simulink model "gm_uz_pmsm_model_9ph_21b_all_double"  (R2021b)
settings: Solver=FixedStepDiscrete  StartTime=0.0  StopTime=0.8  RelTol=1e-3
PreLoadFcn:
  | uz_pmsm_model_9ph_init_parameter
undefined symbols (not defined in the file or in its folder): a, b, c, friction_coefficient, inertia, k_i_d, k_i_q, k_p_d, k_p_q, Kpd, L_d, L_o1, L_o2, L_q, L_x1, L_x2, L_y1, L_y2, L_zero, polepair, psi_pm, R_1, static_friction_torque, Tnd
libraries: hdlmdlgenlib x139, hdlsllib x90, dspsigops x21, simulink x3, slpidlib x2, spsAlphaBetaZerotodq0Lib x1, pid_lib x1, spsdq0toAlphaBetaZeroLib x1
(part 1 of 5)
settings Model: Creator=ts  LastModifiedBy=ts
settings SolverCC: AlgebraicLoopSolver=TrustRegion  AutoInsertRateTranBlk=on
settings DataIOCC: LimitDataPoints=on  SaveOutput=off  SaveTime=off
settings OptimizationCC: BlockReduction=off  ConditionallyExecuteInputs=off  DefaultParameterBehavior=Inlined  InheritOutputTypeSmallerThanSingle=on  LifeSpan=inf
settings DebuggingCC: AlgebraicLoopMsg=error  ArtificialAlgebraicLoopMsg=none  InheritedTsInSrcMsg=none  SingleTaskRateTransMsg=error  AllowSymbolicDim=off  StrictBusMsg=ErrorOnBusTreatedAsVector  SFUnexpectedBacktrackingDiag=warning  SFNoUnconditionalDefaultTransitionDiag=warning  SFExecutionAtInitializationDiag=none  SFMachineParentedDataDiag=warning  ArithmeticOperatorsInVariantConditions=warning
settings HardwareCC: ProdBitPerPointer=32  ProdBitPerSizeT=32  ProdBitPerPtrDiffT=32  ProdLargestAtomicFloat=None  ProdIntDivRoundTo=Undefined  ProdEndianess=Unspecified  ProdWordSize=32  ProdHWDeviceType=ASIC/FPGA->ASIC/FPGA  ProdEqTarget=off
settings SFSimCC: SimUseLocalCustomCode=off  CustomCodeUndefinedFunction=UseInterfaceOnly
settings RTWCC: RTWUseLocalCustomCode=off
settings CodeAppCC: StateflowObjectComments=on
settings GRTTargetCC: TargetLangStandard=C89/C90 (ANSI)
settings ConfigComp: CovScope=ReferencedModels  CovMetricSettings=dw  CovSaveCumulativeToWorkspaceVar=on  CovSaveSingleToWorkspaceVar=on  CovExternalEMLEnable=off  CovSFcnEnable=off

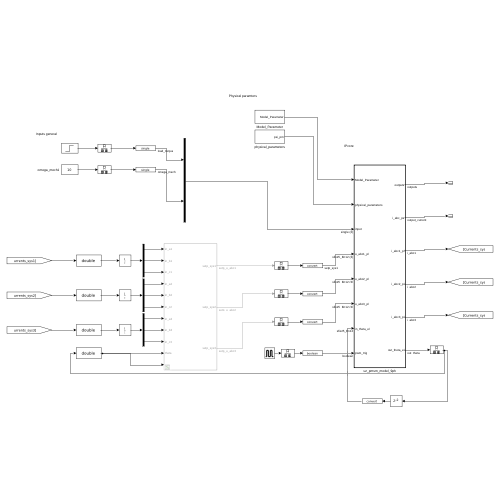
[thumbnail: Simulink's stored preview of the top-level diagram]
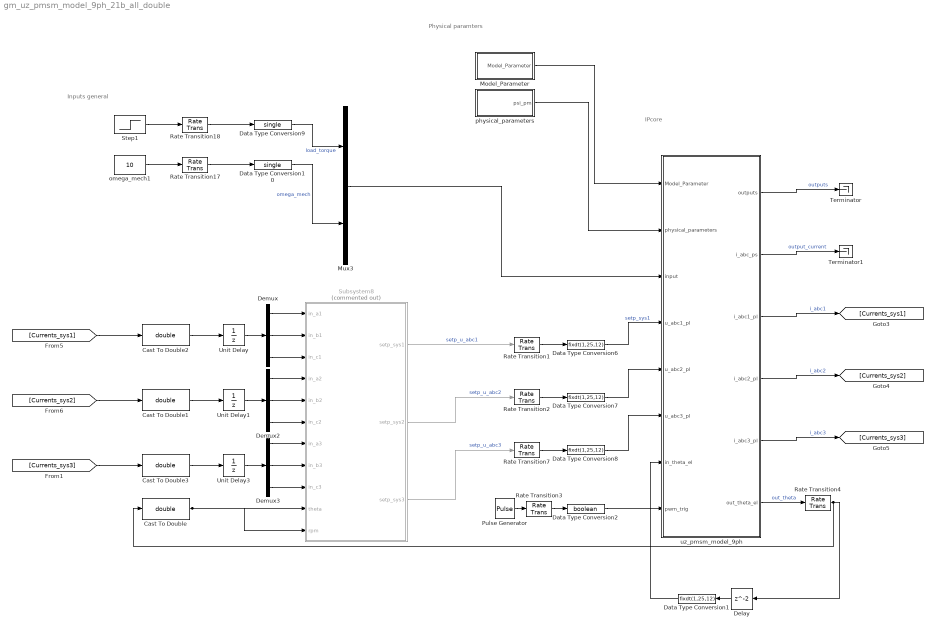
== system gm_uz_pmsm_model_9ph_21b_all_double ==
  note: Inputs general
  note: Physical paramters
  note: IPcore
  Cast To Double{,1..3} (4 alike) : DataTypeConversion  OutDataTypeStr=double
  Data Type Conversion{1,6..8} (4 alike) : DataTypeConversion  OutDataTypeStr=fixdt(1,25,12)  RndMeth=Nearest
  Data Type Conversion10 : DataTypeConversion  OutDataTypeStr=single  RndMeth=Nearest
  Data Type Conversion2 : DataTypeConversion  OutDataTypeStr=boolean  RndMeth=Nearest
  Data Type Conversion9 : DataTypeConversion  OutDataTypeStr=single  RndMeth=Nearest
  Delay : Delay
  Demux : Demux  Outputs=3
  Demux2 : Demux  Outputs=3
  Demux3 : Demux  Outputs=3
  Model_Parameter : Subsystem
  Mux3 : Mux  Inputs=2
  Pulse Generator : DiscretePulseGenerator  PulseType=Time based  Period=1e-9  PulseWidth=50
  Rate Transition{1..4,7,17..18} (7 alike) : RateTransition  OutPortSampleTime=ts
  Step1 : Step  Time=0.25  After=20  SampleTime=0
  Subsystem8 : Subsystem  Commented=on
  Terminator : Terminator
  Terminator1 : Terminator
  Unit Delay : UnitDelay  SampleTime=-1  HasFrameUpgradeWarning=on
  Unit Delay1 : UnitDelay  SampleTime=-1  HasFrameUpgradeWarning=on
  Unit Delay3 : UnitDelay  SampleTime=-1  HasFrameUpgradeWarning=on
  omega_mech1 : Constant  Value=10
  physical_parameters : Subsystem
  uz_pmsm_model_9ph : Subsystem  TreatAsAtomicUnit=on
  wires:
  Rate Transition4/1 -> Cast To Double/1, Delay/1
  Pulse Generator/1 -> Rate Transition3/1
  Rate Transition3/1 -> Data Type Conversion2/1
  Data Type Conversion2/1 -> uz_pmsm_model_9ph/8(pwm_trig)
  Rate Transition7/1 -> Data Type Conversion8/1
  Rate Transition2/1 -> Data Type Conversion7/1
  Rate Transition1/1 -> Data Type Conversion6/1
  Cast To Double3/1 -> Unit Delay3/1
  Cast To Double2/1 -> Unit Delay/1
  Cast To Double1/1 -> Unit Delay1/1
  Cast To Double/1 -> Subsystem8/10(theta), Subsystem8/11(rpm)
  Demux2/3 -> Subsystem8/6(in_c2)
  Demux2/2 -> Subsystem8/5(in_b2)
  Demux/1 -> Subsystem8/1(in_a1)
  Demux3/1 -> Subsystem8/7(in_a3)
  [Currents_sys3] -> Cast To Double3/1
  Unit Delay/1 -> Demux/1
  Demux3/3 -> Subsystem8/9(in_c3)
  [Currents_sys2] -> Cast To Double1/1
  [Currents_sys1] -> Cast To Double2/1
  Demux/3 -> Subsystem8/3(in_c1)
  Unit Delay1/1 -> Demux2/1
  Demux3/2 -> Subsystem8/8(in_b3)
  Demux2/1 -> Subsystem8/4(in_a2)
  Demux/2 -> Subsystem8/2(in_b1)
  Unit Delay3/1 -> Demux3/1
  Data Type Conversion7/1 -> uz_pmsm_model_9ph/5(u_abc2_pl)
  Data Type Conversion8/1 -> uz_pmsm_model_9ph/6(u_abc3_pl)
  Subsystem8/3(setp_sys3) -> Rate Transition7/1  "setp_u_abc3"
  Subsystem8/2(setp_sys2) -> Rate Transition2/1  "setp_u_abc2"
  Data Type Conversion6/1 -> uz_pmsm_model_9ph/4(u_abc1_pl)  "setp_sys1"
  Subsystem8/1(setp_sys1) -> Rate Transition1/1  "setp_u_abc1"
  Delay/1 -> Data Type Conversion1/1
  uz_pmsm_model_9ph/6(out_theta_el) -> Rate Transition4/1  "out_theta"
  uz_pmsm_model_9ph/4(i_abc2_pl) -> [Currents_sys2]  "i_abc2"
  uz_pmsm_model_9ph/5(i_abc3_pl) -> [Currents_sys3]  "i_abc3"
  uz_pmsm_model_9ph/3(i_abc1_pl) -> [Currents_sys1]  "i_abc1"
  uz_pmsm_model_9ph/2(i_abc_ps) -> Terminator1/1  "output_current"
  Data Type Conversion1/1 -> uz_pmsm_model_9ph/7(in_theta_el)
  Mux3/1 -> uz_pmsm_model_9ph/3(input)
  Data Type Conversion9/1 -> Mux3/1  "load_torque"
  Rate Transition17/1 -> Data Type Conversion10/1
  Data Type Conversion10/1 -> Mux3/2  "omega_mech"
  Step1/1 -> Rate Transition18/1
  Rate Transition18/1 -> Data Type Conversion9/1
  omega_mech1/1 -> Rate Transition17/1
  Model_Parameter/1(Model_Parameter) -> uz_pmsm_model_9ph/1(Model_Parameter)
  uz_pmsm_model_9ph/1(outputs) -> Terminator/1  "outputs"
  physical_parameters/1(psi_pm) -> uz_pmsm_model_9ph/2(physical_parameters)

== system gm_uz_pmsm_model_9ph_21b_all_double/Model_Parameter ==
  note: This flag determines if omega_mech is used as an input value or
      | if the mechanical system is simulated by the model
  Bus Creator : BusCreator  Inputs=4
  Constant3 : Constant  Value=0
  Data Type Conversion{3..4,9..10} (4 alike) : DataTypeConversion  OutDataTypeStr=boolean
  Rate Transition{6,8,17..18} (4 alike) : RateTransition  OutPortSampleTime=ts
  simulate_mechanical : Constant  Value=false
  simulate_mechanical1 : Constant  Value=false
  simulate_mechanical2 : Constant  Value=false
  Model_Parameter : Outport
  wires:
  Data Type Conversion3/1 -> Bus Creator/1  "reset_integrators"
  Bus Creator/1 -> Model_Parameter/1
  Data Type Conversion4/1 -> Bus Creator/2  "simulate_mechanical"
  Data Type Conversion9/1 -> Bus Creator/3  "switch_pspl"
  Data Type Conversion10/1 -> Bus Creator/4  "control_dq_abc"
  Rate Transition18/1 -> Data Type Conversion10/1
  Rate Transition17/1 -> Data Type Conversion9/1
  simulate_mechanical1/1 -> Rate Transition17/1
  Constant3/1 -> Rate Transition6/1
  Rate Transition6/1 -> Data Type Conversion3/1
  Rate Transition8/1 -> Data Type Conversion4/1
  simulate_mechanical/1 -> Rate Transition8/1
  simulate_mechanical2/1 -> Rate Transition18/1

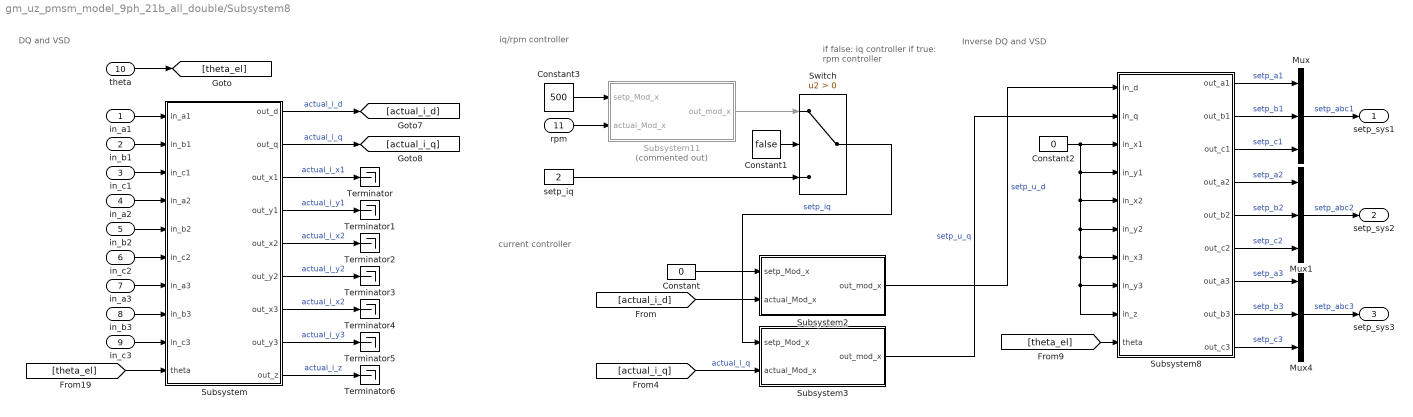
== system gm_uz_pmsm_model_9ph_21b_all_double/Subsystem8 ==
  note: Inverse DQ and VSD
  note: if false: iq controller
      | if true: rpm controller
  note: iq/rpm controller
  note: current controller
  note: DQ and VSD
  in_a1 : Inport
  in_b1 : Inport  Port=2
  in_c1 : Inport  Port=3
  in_a2 : Inport  Port=4
  in_b2 : Inport  Port=5
  in_c2 : Inport  Port=6
  in_a3 : Inport  Port=7
  in_b3 : Inport  Port=8
  in_c3 : Inport  Port=9
  theta : Inport  Port=10
  rpm : Inport  Port=11
  Constant : Constant  Value=0
  Constant1 : Constant  Value=false
  Constant2 : Constant  Value=0
  Constant3 : Constant  Value=500
  Mux : Mux  Inputs=3
  Mux1 : Mux  Inputs=3
  Mux4 : Mux  Inputs=3
  Subsystem : Subsystem
  Subsystem11 : Subsystem  Commented=on
  Subsystem2 : Subsystem
  Subsystem3 : Subsystem
  Subsystem8 : Subsystem
  Switch : Switch  Criteria=u2 > Threshold
  Terminator{,1..6} (7 alike) : Terminator
  setp_iq : Constant  Value=2
  setp_sys1 : Outport
  setp_sys2 : Outport  Port=2
  setp_sys3 : Outport  Port=3
  wires:
  Subsystem2/1(out_mod_x) -> Subsystem8/1(in_d)  "setp_u_d"
  Subsystem3/1(out_mod_x) -> Subsystem8/2(in_q)  "setp_u_q"
  Constant3/1 -> Subsystem11/1(setp_Mod_x)
  setp_iq/1 -> Switch/3
  Constant1/1 -> Switch/2
  Switch/1 -> Subsystem3/1(setp_Mod_x)  "setp_iq"
  Subsystem11/1(out_mod_x) -> Switch/1
  Constant2/1 -> Subsystem8/4(in_y1), Subsystem8/5(in_x2), Subsystem8/6(in_y2), Subsystem8/7(in_x3), Subsystem8/9(in_z), Subsystem8/8(in_y3), Subsystem8/3(in_x1)
  [theta_el] -> Subsystem/10(theta)
  Subsystem/2(out_q) -> [actual_i_q]  "actual_i_q"
  Subsystem/1(out_d) -> [actual_i_d]  "actual_i_d"
  rpm/1 -> Subsystem11/2(actual_Mod_x)
  Subsystem8/9(out_c3) -> Mux4/3  "setp_c3"
  Subsystem8/8(out_b3) -> Mux4/2  "setp_b3"
  Subsystem8/7(out_a3) -> Mux4/1  "setp_a3"
  Mux4/1 -> setp_sys3/1  "setp_abc3"
  Subsystem8/4(out_a2) -> Mux1/1  "setp_a2"
  Subsystem8/5(out_b2) -> Mux1/2  "setp_b2"
  Subsystem8/6(out_c2) -> Mux1/3  "setp_c2"
  Mux1/1 -> setp_sys2/1  "setp_abc2"
  in_a3/1 -> Subsystem/7(in_a3)
  in_b3/1 -> Subsystem/8(in_b3)
  in_c3/1 -> Subsystem/9(in_c3)
  Subsystem/9(out_z) -> Terminator6/1  "actual_i_z"
  Subsystem/7(out_x3) -> Terminator4/1  "actual_i_x2"
  Subsystem/8(out_y3) -> Terminator5/1  "actual_i_y3"
  Mux/1 -> setp_sys1/1  "setp_abc1"
  theta/1 -> [theta_el]
  in_c2/1 -> Subsystem/6(in_c2)
  in_a2/1 -> Subsystem/4(in_a2)
  in_b2/1 -> Subsystem/5(in_b2)
  [actual_i_q] -> Subsystem3/2(actual_Mod_x)  "actual_i_q"
  in_a1/1 -> Subsystem/1(in_a1)
  Subsystem/5(out_x2) -> Terminator2/1  "actual_i_x2"
  Subsystem/6(out_y2) -> Terminator3/1  "actual_i_y2"
  Constant/1 -> Subsystem2/1(setp_Mod_x)
  [actual_i_d] -> Subsystem2/2(actual_Mod_x)
  in_c1/1 -> Subsystem/3(in_c1)
  Subsystem/3(out_x1) -> Terminator/1  "actual_i_x1"
  Subsystem8/3(out_c1) -> Mux/3  "setp_c1"
  Subsystem8/2(out_b1) -> Mux/2  "setp_b1"
  [theta_el] -> Subsystem8/10(theta)
  in_b1/1 -> Subsystem/2(in_b1)
  Subsystem8/1(out_a1) -> Mux/1  "setp_a1"
  Subsystem/4(out_y1) -> Terminator1/1  "actual_i_y1"

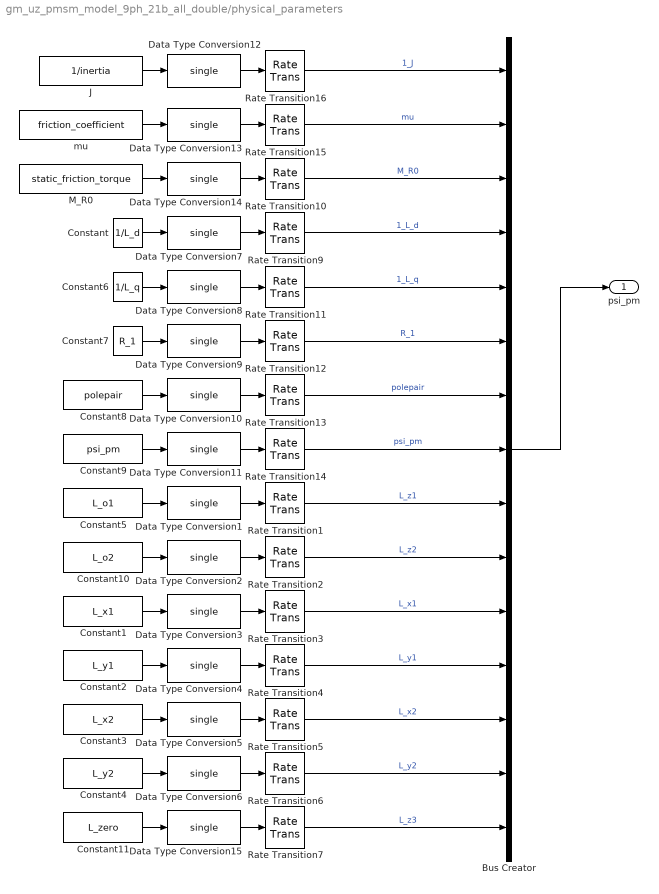
== system gm_uz_pmsm_model_9ph_21b_all_double/physical_parameters ==
  Bus Creator : BusCreator  Inputs=15
  Constant : Constant  Value=1/L_d
  Constant1 : Constant  Value=L_x1
  Constant10 : Constant  Value=L_o2
  Constant11 : Constant  Value=L_zero
  Constant2 : Constant  Value=L_y1
  Constant3 : Constant  Value=L_x2
  Constant4 : Constant  Value=L_y2
  Constant5 : Constant  Value=L_o1
  Constant6 : Constant  Value=1/L_q
  Constant7 : Constant  Value=R_1
  Constant8 : Constant  Value=polepair
  Constant9 : Constant  Value=psi_pm
  Data Type Conversion{1..15} (15 alike) : DataTypeConversion  OutDataTypeStr=single
  J : Constant  Value=1/inertia
  M_R0 : Constant  Value=static_friction_torque
  Rate Transition{1..7,9..16} (15 alike) : RateTransition  OutPortSampleTime=ts
  mu : Constant  Value=friction_coefficient
  psi_pm : Outport
  wires:
  Constant10/1 -> Data Type Conversion2/1
  Constant5/1 -> Data Type Conversion1/1
  Constant1/1 -> Data Type Conversion3/1
  Constant2/1 -> Data Type Conversion4/1
  Constant3/1 -> Data Type Conversion5/1
  Constant4/1 -> Data Type Conversion6/1
  Rate Transition2/1 -> Bus Creator/10  "L_z2"
  Rate Transition3/1 -> Bus Creator/11  "L_x1"
  Rate Transition4/1 -> Bus Creator/12  "L_y1"
  Rate Transition5/1 -> Bus Creator/13  "L_x2"
  Rate Transition6/1 -> Bus Creator/14  "L_y2"
  Rate Transition7/1 -> Bus Creator/15  "L_z3"
  Rate Transition1/1 -> Bus Creator/9  "L_z1"
  Data Type Conversion15/1 -> Rate Transition7/1
  Constant11/1 -> Data Type Conversion15/1
  Data Type Conversion6/1 -> Rate Transition6/1
  Data Type Conversion5/1 -> Rate Transition5/1
  Data Type Conversion4/1 -> Rate Transition4/1
  Data Type Conversion3/1 -> Rate Transition3/1
  Data Type Conversion2/1 -> Rate Transition2/1
  Data Type Conversion1/1 -> Rate Transition1/1
  Constant/1 -> Data Type Conversion7/1
  Constant9/1 -> Data Type Conversion11/1
  Constant7/1 -> Data Type Conversion9/1
  Data Type Conversion13/1 -> Rate Transition15/1
  Rate Transition11/1 -> Bus Creator/5  "1_L_q"
  M_R0/1 -> Data Type Conversion14/1
  mu/1 -> Data Type Conversion13/1
  Data Type Conversion10/1 -> Rate Transition13/1
  Data Type Conversion8/1 -> Rate Transition11/1
  J/1 -> Data Type Conversion12/1
  Rate Transition9/1 -> Bus Creator/4  "1_L_d"
  Constant6/1 -> Data Type Conversion8/1
  Rate Transition15/1 -> Bus Creator/2  "mu"
  Data Type Conversion9/1 -> Rate Transition12/1
  Constant8/1 -> Data Type Conversion10/1
  Data Type Conversion11/1 -> Rate Transition14/1
  Bus Creator/1 -> psi_pm/1
  Rate Transition13/1 -> Bus Creator/7  "polepair"
  Rate Transition16/1 -> Bus Creator/1  "1_J"
  Rate Transition12/1 -> Bus Creator/6  "R_1"
  Data Type Conversion14/1 -> Rate Transition10/1
  Rate Transition14/1 -> Bus Creator/8  "psi_pm"
  Rate Transition10/1 -> Bus Creator/3  "M_R0"
  Data Type Conversion7/1 -> Rate Transition9/1
  Data Type Conversion12/1 -> Rate Transition16/1

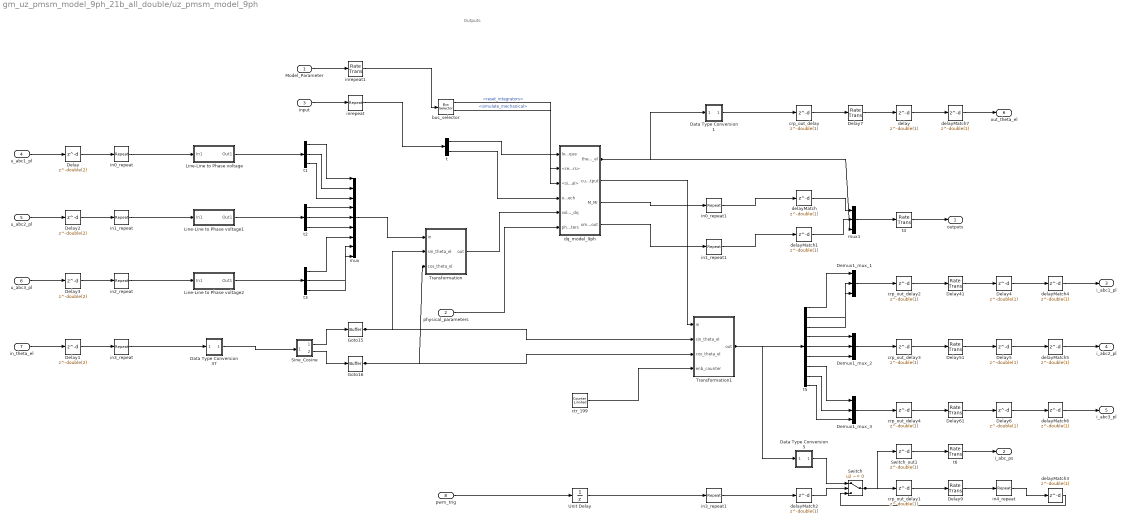
== system gm_uz_pmsm_model_9ph_21b_all_double/uz_pmsm_model_9ph ==
  note: Outputs
  Model_Parameter : Inport  SampleTime=2e-06
  physical_parameters : Inport  Port=2  SampleTime=2e-06
  input : Inport  Port=3  OutDataTypeStr=single  PortDimensions=[2]  SampleTime=2e-06
  u_abc1_pl : Inport  Port=4  OutDataTypeStr=fixdt(1, 25, 12)  PortDimensions=[3]  SampleTime=2e-06
  u_abc2_pl : Inport  Port=5  OutDataTypeStr=fixdt(1, 25, 12)  PortDimensions=[3]  SampleTime=2e-06
  u_abc3_pl : Inport  Port=6  OutDataTypeStr=fixdt(1, 25, 12)  PortDimensions=[3]  SampleTime=2e-06
  in_theta_el : Inport  Port=7  OutDataTypeStr=fixdt(1, 25, 12)  PortDimensions=1  SampleTime=2e-06
  pwm_trig : Inport  Port=8  OutDataTypeStr=boolean  PortDimensions=1  SampleTime=2e-06
  Data Type Conversion1 : Subsystem
      mask Display: disp('NFP\nconv');
  Data Type Conversion37 : Subsystem
      mask Display: disp('NFP\nconv');
  Data Type Conversion5 : Subsystem
      mask Display: disp('NFP\nconv');
  Delay{,1..3} (4 alike) : Delay  DelayLength=double(2)  InitialCondition=0  SampleTime=2e-06
  Delay4 : Delay  DelayLength=double(1)  InitialCondition=0  SampleTime=2e-06
  Delay{7,9,41,51,61} (5 alike) : RateTransition  OutPortSampleTimeOpt=Multiple of input port sample time  OutPortSampleTimeMultiple=200
  Delay5 : Delay  DelayLength=double(1)  InitialCondition=0  SampleTime=2e-06
  Delay6 : Delay  DelayLength=double(1)  InitialCondition=0  SampleTime=2e-06
  Demux1_mux_1 : Mux  Inputs=3
  Demux1_mux_2 : Mux  Inputs=3
  Demux1_mux_3 : Mux  Inputs=3
  Goto15 : hdlmdlgenlib/Buffer
      settings: SourceProductBaseCode=SL
  Goto16 : hdlmdlgenlib/Buffer
      settings: SourceProductBaseCode=SL
  Line-Line to Phase voltage : Subsystem
  Line-Line to Phase voltage1 : Subsystem
  Line-Line to Phase voltage2 : Subsystem
  Sine_Cosine : Subsystem
      mask Display: disp('NFP\ntrig2');
  Switch : Switch  Criteria=u2 ~= 0  Threshold=double(0)  OutDataTypeStr=single  SampleTime=1e-08
  Switch_out1 : Delay  DelayLength=double(1)  InitialCondition=0  SampleTime=1e-08
  Transformation : Subsystem
  Transformation1 : Subsystem
  Unit Delay : UnitDelay  SampleTime=2e-06
  bus_selector : BusSelector  OutputSignals=reset_integrators,simulate_mechanical
  crp_out_delay{,1..4} (5 alike) : Delay  DelayLength=double(1)  InitialCondition=0  SampleTime=1e-08
  ctr_199 : simulink/Sources/Counter Limited  uplimit=double(199)  tsamp=1e-08
  delay : Delay  DelayLength=double(1)  InitialCondition=0  SampleTime=2e-06
  delayMatch{,1..3} (4 alike) : Delay  DelayLength=double(1)  InitialCondition=0  SampleTime=1e-08
  delayMatch{4..7} (4 alike) : Delay  DelayLength=double(1)  InitialCondition=0  SampleTime=2e-06
  dq_model_9ph : Subsystem
  in0_repeat : dspsigops/Repeat  N=double(200)  RateOptions=Allow multirate processing  ic=0  mode=Unused parameter value
  in0_repeat1 : dspsigops/Repeat  N=double(200)  RateOptions=Allow multirate processing  ic=0  mode=Unused parameter value
  in1_repeat : dspsigops/Repeat  N=double(200)  RateOptions=Allow multirate processing  ic=0  mode=Unused parameter value
  in1_repeat1 : dspsigops/Repeat  N=double(200)  RateOptions=Allow multirate processing  ic=0  mode=Unused parameter value
  in2_repeat : dspsigops/Repeat  N=double(200)  RateOptions=Allow multirate processing  ic=0  mode=Unused parameter value
  in3_repeat : dspsigops/Repeat  N=double(200)  RateOptions=Allow multirate processing  ic=0  mode=Unused parameter value
  in3_repeat1 : dspsigops/Repeat  N=double(200)  RateOptions=Allow multirate processing  ic=0  mode=Unused parameter value
  in4_repeat : dspsigops/Repeat  N=double(200)  RateOptions=Allow multirate processing  ic=0  mode=Unused parameter value
  inrepeat : dspsigops/Repeat  N=double(200)  RateOptions=Allow multirate processing  ic=0  mode=Unused parameter value
  inrepeat1 : RateTransition  Integrity=off  Deterministic=off  OutPortSampleTimeOpt=Multiple of input port sample time  OutPortSampleTimeMultiple=1/200
  mux : Mux  Inputs=9
  mux1 : Mux  Inputs=3
  t : Demux  Outputs=2
  t1 : Demux  Outputs=3
  t2 : Demux  Outputs=3
  t3 : Demux  Outputs=3
  t4 : RateTransition  OutPortSampleTimeOpt=Multiple of input port sample time  OutPortSampleTimeMultiple=200
  t5 : Demux  Outputs=9
  t6 : RateTransition  OutPortSampleTimeOpt=Multiple of input port sample time  OutPortSampleTimeMultiple=200
  outputs : Outport  SampleTime=2e-06
  i_abc_ps : Outport  Port=2  SampleTime=2e-06
  i_abc1_pl : Outport  Port=3  SampleTime=2e-06
  i_abc2_pl : Outport  Port=4  SampleTime=2e-06
  i_abc3_pl : Outport  Port=5  SampleTime=2e-06
  out_theta_el : Outport  Port=6  SampleTime=2e-06
  wires:
  Model_Parameter/1 -> inrepeat1/1
  physical_parameters/1 -> dq_model_9ph/6(physical_parameters)
  input/1 -> inrepeat/1
  u_abc1_pl/1 -> Delay/1
  u_abc2_pl/1 -> Delay2/1
  u_abc3_pl/1 -> Delay3/1
  in_theta_el/1 -> Delay1/1
  pwm_trig/1 -> Unit Delay/1
  delayMatch7/1 -> out_theta_el/1
  Delay/1 -> in0_repeat/1
  Delay1/1 -> in3_repeat/1
  Delay2/1 -> in1_repeat/1
  Delay3/1 -> in2_repeat/1
  delayMatch4/1 -> i_abc1_pl/1
  delayMatch5/1 -> i_abc2_pl/1
  delayMatch6/1 -> i_abc3_pl/1
  Delay41/1 -> Delay4/1
  Delay51/1 -> Delay5/1
  Delay61/1 -> Delay6/1
  Unit Delay/1 -> in3_repeat1/1
  dq_model_9ph/3(M_Mi) -> in0_repeat1/1
  dq_model_9ph/4(omega_out) -> in1_repeat1/1
  Delay7/1 -> delay/1
  t/1 -> dq_model_9ph/1(load_torque)
  t/2 -> dq_model_9ph/4(omega_mech)
  bus_selector/1 -> dq_model_9ph/2(<reset_integrators>)  "<reset_integrators>"
  bus_selector/2 -> dq_model_9ph/3(<simulate_mechanical>)  "<simulate_mechanical>"
  Goto15/1 -> Transformation/2(sin_theta_el), Transformation1/2(sin_theta_el)
  Goto16/1 -> Transformation/3(cos_theta_el), Transformation1/3(cos_theta_el)
  Transformation/1(out) -> dq_model_9ph/5(voltage_input_dq)
  dq_model_9ph/1(theta_el) -> mux1/3, Data Type Conversion1/1(In1)
  dq_model_9ph/2(currents_dq_output) -> Transformation1/1(in)
  t4/1 -> outputs/1
  t6/1 -> i_abc_ps/1
  Delay4/1 -> delayMatch4/1
  Delay5/1 -> delayMatch5/1
  Delay6/1 -> delayMatch6/1
  delay/1 -> delayMatch7/1
  Delay9/1 -> in4_repeat/1
  inrepeat/1 -> t/1
  inrepeat1/1 -> bus_selector/1
  in0_repeat/1 -> Line-Line to Phase voltage/1(In1)
  in1_repeat/1 -> Line-Line to Phase voltage1/1(In1)
  in2_repeat/1 -> Line-Line to Phase voltage2/1(In1)
  in3_repeat/1 -> Data Type Conversion37/1(In1)
  Line-Line to Phase voltage/1(Out1) -> t1/1
  Line-Line to Phase voltage1/1(Out1) -> t2/1
  Line-Line to Phase voltage2/1(Out1) -> t3/1
  t1/1 -> mux/1
  t1/2 -> mux/2
  t1/3 -> mux/3
  t2/1 -> mux/4
  t2/2 -> mux/5
  t2/3 -> mux/6
  t3/1 -> mux/7
  t3/2 -> mux/8
  t3/3 -> mux/9
  Data Type Conversion37/1(Out1) -> Sine_Cosine/1(In1)
  Sine_Cosine/1(Out1) -> Goto15/1
  Sine_Cosine/2(Out2) -> Goto16/1
  mux/1 -> Transformation/1(in)
  mux1/1 -> t4/1
  in0_repeat1/1 -> delayMatch/1
  in1_repeat1/1 -> delayMatch1/1
  delayMatch/1 -> mux1/1
  delayMatch1/1 -> mux1/2
  crp_out_delay/1 -> Delay7/1
  Data Type Conversion1/1(Out1) -> crp_out_delay/1
  Switch_out1/1 -> t6/1
  crp_out_delay1/1 -> Delay9/1
  crp_out_delay2/1 -> Delay41/1
  crp_out_delay3/1 -> Delay51/1
  crp_out_delay4/1 -> Delay61/1
  in3_repeat1/1 -> delayMatch2/1
  in4_repeat/1 -> delayMatch3/1
  Transformation1/1(out) -> Data Type Conversion5/1(In1), t5/1
  t5/1 -> Demux1_mux_1/1
  t5/2 -> Demux1_mux_1/2
  t5/3 -> Demux1_mux_1/3
  t5/4 -> Demux1_mux_2/1
  t5/5 -> Demux1_mux_2/2
  t5/6 -> Demux1_mux_2/3
  t5/7 -> Demux1_mux_3/1
  t5/8 -> Demux1_mux_3/2
  t5/9 -> Demux1_mux_3/3
  delayMatch2/1 -> Switch/2
  delayMatch3/1 -> Switch/3
  Data Type Conversion5/1(Out1) -> Switch/1
  Demux1_mux_1/1 -> crp_out_delay2/1
  Demux1_mux_2/1 -> crp_out_delay3/1
  Demux1_mux_3/1 -> crp_out_delay4/1
  Switch/1 -> crp_out_delay1/1, Switch_out1/1
  ctr_199/1 -> Transformation1/4(enb_counter)

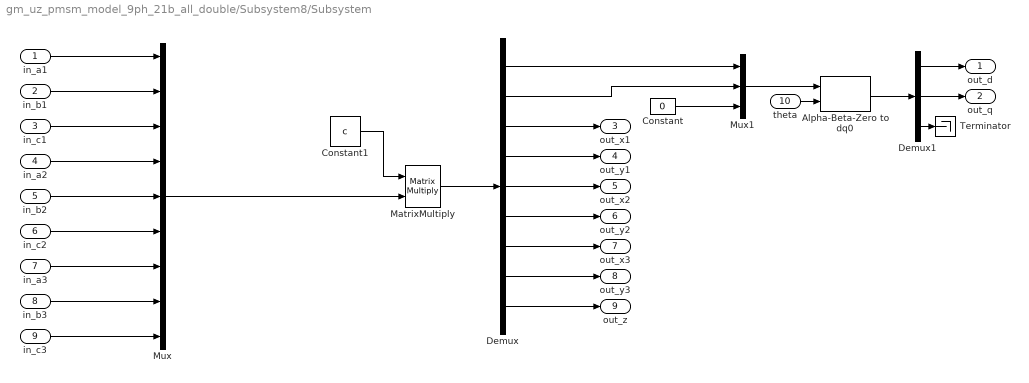
== system gm_uz_pmsm_model_9ph_21b_all_double/Subsystem8/Subsystem ==
  in_a1 : Inport
  in_b1 : Inport  Port=2
  in_c1 : Inport  Port=3
  in_a2 : Inport  Port=4
  in_b2 : Inport  Port=5
  in_c2 : Inport  Port=6
  in_a3 : Inport  Port=7
  in_b3 : Inport  Port=8
  in_c3 : Inport  Port=9
  theta : Inport  Port=10
  Alpha-Beta-Zero to dq0 : spsAlphaBetaZerotodq0Lib/Alpha-Beta-Zero to dq0  Alignment=90 degrees behind phase A axis
      settings: SourceProductBaseCode=PS
  Constant : Constant  Value=0
  Constant1 : Constant  Value=c
  Demux : Demux  Outputs=9
  Demux1 : Demux  Outputs=3
  MatrixMultiply : Product  Multiplication=Matrix(*)
  Mux : Mux  Inputs=9
  Mux1 : Mux  Inputs=3
  Terminator : Terminator
  out_d : Outport
  out_q : Outport  Port=2
  out_x1 : Outport  Port=3
  out_y1 : Outport  Port=4
  out_x2 : Outport  Port=5
  out_y2 : Outport  Port=6
  out_x3 : Outport  Port=7
  out_y3 : Outport  Port=8
  out_z : Outport  Port=9
  wires:
  in_b3/1 -> Mux/8
  in_a3/1 -> Mux/7
  in_c2/1 -> Mux/6
  in_b2/1 -> Mux/5
  in_a2/1 -> Mux/4
  in_c1/1 -> Mux/3
  in_b1/1 -> Mux/2
  Mux/1 -> MatrixMultiply/2
  Constant1/1 -> MatrixMultiply/1
  Alpha-Beta-Zero to dq0/1 -> Demux1/1
  Constant/1 -> Mux1/3
  Demux1/2 -> out_q/1
  Demux1/1 -> out_d/1
  Demux/2 -> Mux1/2
  Mux1/1 -> Alpha-Beta-Zero to dq0/1
  Demux/1 -> Mux1/1
  Demux1/3 -> Terminator/1
  theta/1 -> Alpha-Beta-Zero to dq0/2
  Demux/9 -> out_z/1
  Demux/8 -> out_y3/1
  Demux/7 -> out_x3/1
  in_c3/1 -> Mux/9
  Demux/3 -> out_x1/1
  MatrixMultiply/1 -> Demux/1
  Demux/5 -> out_x2/1
  in_a1/1 -> Mux/1
  Demux/4 -> out_y1/1
  Demux/6 -> out_y2/1

== system gm_uz_pmsm_model_9ph_21b_all_double/Subsystem8/Subsystem11 ==
  setp_Mod_x : Inport
  actual_Mod_x : Inport  Port=2
  Add : Sum  Inputs=+-
  Data Type Conversion8 : DataTypeConversion  OutDataTypeStr=double
  PID Controller2 : pid_lib/PID Controller  Controller=PI  Form=Ideal  TimeDomain=Continuous-time  UseExternalTs=off  SampleTime=-1  IntegratorMethod=Forward Euler  FilterMethod=Forward Euler  ControllerParametersSource=internal  P=Kpd  I=1/Tnd  D=0  N=100  UseFilter=on  TunerSelectOption=Transfer Function Based (PID Tuner App)  InitialConditionSource=internal  InitialConditionForIntegrator=0  InitialConditionForFilter=0  DifferentiatorICPrevScaledInput=0  ExternalReset=none  TrackingMode=off  Kt=1  LimitOutput=on  SatLimitsSource=internal  UpperSaturationLimit=50  LowerSaturationLimit=-50  LinearizeAsGain=on  AntiWindupMode=clamping  Kb=1  POutMin=[]  POutMax=[]  IOutMin=[]  IOutMax=[]  DOutMin=[]  DOutMax=[]  NOutMin=[]  NOutMax=[]  SumOutMin=[]  SumOutMax=[]  SaturationOutMin=[]  SaturationOutMax=[]  PParamMin=[]  PParamMax=[]  IParamMin=[]  IParamMax=[]  DParamMin=[]  DParamMax=[]  NParamMin=[]  NParamMax=[]  KbParamMin=[]  KbParamMax=[]  KtParamMin=[]  KtParamMax=[]  KbOutMin=[]  KbOutMax=[]  KtOutMin=[]  KtOutMax=[]  IntegratorOutMin=[]  IntegratorOutMax=[]  FilterOutMin=[]  FilterOutMax=[]  SumI1OutMin=[]  SumI1OutMax=[]  SumI2OutMin=[]  SumI2OutMax=[]  SumI3OutMin=[]  SumI3OutMax=[]  SumI4OutMin=[]  SumI4OutMax=[]  SumDOutMin=[]  SumDOutMax=[]  DifferentiatorOutMin=[]  DifferentiatorOutMax=[]  FilterDiffOutCoefMin=[]  FilterDiffOutCoefMax=[]  ReciprocalOutMin=[]  ReciprocalOutMax=[]  SumDenOutMin=[]  SumDenOutMax=[]  SumNumOutMin=[]  SumNumOutMax=[]  DivideOutMin=[]  DivideOutMax=[]  UdiffTsProdOutMin=[]  UdiffTsProdOutMax=[]  NTsProdOutMin=[]  NTsProdOutMax=[]  UintegralTsProdOutMin=[]  UintegralTsProdOutMax=[]  UngainTsProdOutMin=[]  UngainTsProdOutMax=[]  IntegratorContinuousStateAttributes=''  IntegratorStateMustResolveToSignalObject=off  IntegratorRTWStateStorageClass=Auto  FilterContinuousStateAttributes=''  FilterStateMustResolveToSignalObject=off  FilterRTWStateStorageClass=Auto  ParallelPVariant=Passthrough  IdealPVariant=InternalParameters  IVariant=InternalParameters  DVariant=Disabled  IntegratorVariant=Continuous  SatVariant=Enabled  AWVariant=ContClampingIdeal  PCopyVariant=InternalParamsIdeal  TRVariant=Disabled  FdbkBlocksVariant=Forward  IdealPFdbkVariant=Disabled  SatFdbkVariant=Disabled  DerivativeFilterVariant=Disabled  NVariant=Disabled  NCopyVariant=Disabled_SignalSpec  FilterICVariant=Disabled  IntegratorICVariant=InternalICs  ExternalResetVariant=Disabled  TRSumVariant=Passthrough  SumFdbkVariant=Disabled  SumVariant=Sum_PI  TsampFilterVariant=InternalTs  TsampNgainVariant=Passthrough  TsampIntegralVariant=Passthrough  ExternalSaturationOutDataTypeStr=Inherit: Same as second input
  out_mod_x : Outport
  wires:
  PID Controller2/1 -> out_mod_x/1
  setp_Mod_x/1 -> Add/1
  Data Type Conversion8/1 -> PID Controller2/1
  actual_Mod_x/1 -> Add/2
  Add/1 -> Data Type Conversion8/1

== system gm_uz_pmsm_model_9ph_21b_all_double/Subsystem8/Subsystem2 ==
  setp_Mod_x : Inport
  actual_Mod_x : Inport  Port=2
  Add : Sum  Inputs=+-
  Data Type Conversion8 : DataTypeConversion  OutDataTypeStr=double
  PID Controller2 : slpidlib/PID Controller  Controller=PI  Form=Ideal  TimeDomain=Continuous-time  UseExternalTs=off  SampleTime=-1  IntegratorMethod=Forward Euler  FilterMethod=Forward Euler  ControllerParametersSource=internal  P=k_p_d  I=k_i_d  D=0  UseFilter=on  N=100  TunerSelectOption=Transfer Function Based (PID Tuner App)  InitialConditionSource=internal  InitialConditionForIntegrator=0  InitialConditionForFilter=0  DifferentiatorICPrevScaledInput=0  ExternalReset=none  TrackingMode=off  Kt=1  LimitOutput=on  SatLimitsSource=internal  UpperSaturationLimit=100  LowerSaturationLimit=-100  LinearizeAsGain=on  AntiWindupMode=clamping  Kb=1  POutMin=[]  POutMax=[]  IOutMin=[]  IOutMax=[]  DOutMin=[]  DOutMax=[]  NOutMin=[]  NOutMax=[]  SumOutMin=[]  SumOutMax=[]  SaturationOutMin=[]  SaturationOutMax=[]  PParamMin=[]  PParamMax=[]  IParamMin=[]  IParamMax=[]  DParamMin=[]  DParamMax=[]  NParamMin=[]  NParamMax=[]  KbParamMin=[]  KbParamMax=[]  KtParamMin=[]  KtParamMax=[]  KbOutMin=[]  KbOutMax=[]  KtOutMin=[]  KtOutMax=[]  IntegratorOutMin=[]  IntegratorOutMax=[]  FilterOutMin=[]  FilterOutMax=[]  SumI1OutMin=[]  SumI1OutMax=[]  SumI2OutMin=[]  SumI2OutMax=[]  SumI3OutMin=[]  SumI3OutMax=[]  SumI4OutMin=[]  SumI4OutMax=[]  SumDOutMin=[]  SumDOutMax=[]  DifferentiatorOutMin=[]  DifferentiatorOutMax=[]  FilterDiffOutCoefMin=[]  FilterDiffOutCoefMax=[]  ReciprocalOutMin=[]  ReciprocalOutMax=[]  SumDenOutMin=[]  SumDenOutMax=[]  SumNumOutMin=[]  SumNumOutMax=[]  DivideOutMin=[]  DivideOutMax=[]  UdiffTsProdOutMin=[]  UdiffTsProdOutMax=[]  NTsProdOutMin=[]  NTsProdOutMax=[]  UintegralTsProdOutMin=[]  UintegralTsProdOutMax=[]  UngainTsProdOutMin=[]  UngainTsProdOutMax=[]  IntegratorContinuousStateAttributes=''  IntegratorStateMustResolveToSignalObject=off  IntegratorRTWStateStorageClass=Auto  FilterContinuousStateAttributes=''  FilterStateMustResolveToSignalObject=off  FilterRTWStateStorageClass=Auto  ParallelPVariant=Passthrough  IdealPVariant=InternalParameters  IVariant=InternalParameters  DVariant=Disabled  IntegratorVariant=Continuous  SatVariant=Enabled  AWVariant=ContClampingIdeal  PCopyVariant=InternalParamsIdeal  TRVariant=Disabled  FdbkBlocksVariant=Forward  IdealPFdbkVariant=Disabled  SatFdbkVariant=Disabled  DerivativeFilterVariant=Disabled  NVariant=Disabled  NCopyVariant=Disabled_SignalSpec  FilterICVariant=Disabled  IntegratorICVariant=InternalICs  ExternalResetVariant=Disabled  TRSumVariant=Passthrough  SumFdbkVariant=Disabled  SumVariant=Sum_PI  TsampFilterVariant=InternalTs  TsampNgainVariant=Passthrough  TsampIntegralVariant=Passthrough  ExternalSaturationOutDataTypeStr=Inherit: Same as second input
  out_mod_x : Outport
  wires:
  PID Controller2/1 -> out_mod_x/1
  setp_Mod_x/1 -> Add/1
  Data Type Conversion8/1 -> PID Controller2/1
  actual_Mod_x/1 -> Add/2
  Add/1 -> Data Type Conversion8/1

== system gm_uz_pmsm_model_9ph_21b_all_double/Subsystem8/Subsystem3 ==
  setp_Mod_x : Inport
  actual_Mod_x : Inport  Port=2
  Add : Sum  Inputs=+-
  Data Type Conversion8 : DataTypeConversion  OutDataTypeStr=double
  PID Controller2 : slpidlib/PID Controller  Controller=PI  Form=Ideal  TimeDomain=Continuous-time  UseExternalTs=off  SampleTime=-1  IntegratorMethod=Forward Euler  FilterMethod=Forward Euler  ControllerParametersSource=internal  P=k_p_q  I=k_i_q  D=0  UseFilter=on  N=100  TunerSelectOption=Transfer Function Based (PID Tuner App)  InitialConditionSource=internal  InitialConditionForIntegrator=0  InitialConditionForFilter=0  DifferentiatorICPrevScaledInput=0  ExternalReset=none  TrackingMode=off  Kt=1  LimitOutput=on  SatLimitsSource=internal  UpperSaturationLimit=100  LowerSaturationLimit=-100  LinearizeAsGain=on  AntiWindupMode=clamping  Kb=1  POutMin=[]  POutMax=[]  IOutMin=[]  IOutMax=[]  DOutMin=[]  DOutMax=[]  NOutMin=[]  NOutMax=[]  SumOutMin=[]  SumOutMax=[]  SaturationOutMin=[]  SaturationOutMax=[]  PParamMin=[]  PParamMax=[]  IParamMin=[]  IParamMax=[]  DParamMin=[]  DParamMax=[]  NParamMin=[]  NParamMax=[]  KbParamMin=[]  KbParamMax=[]  KtParamMin=[]  KtParamMax=[]  KbOutMin=[]  KbOutMax=[]  KtOutMin=[]  KtOutMax=[]  IntegratorOutMin=[]  IntegratorOutMax=[]  FilterOutMin=[]  FilterOutMax=[]  SumI1OutMin=[]  SumI1OutMax=[]  SumI2OutMin=[]  SumI2OutMax=[]  SumI3OutMin=[]  SumI3OutMax=[]  SumI4OutMin=[]  SumI4OutMax=[]  SumDOutMin=[]  SumDOutMax=[]  DifferentiatorOutMin=[]  DifferentiatorOutMax=[]  FilterDiffOutCoefMin=[]  FilterDiffOutCoefMax=[]  ReciprocalOutMin=[]  ReciprocalOutMax=[]  SumDenOutMin=[]  SumDenOutMax=[]  SumNumOutMin=[]  SumNumOutMax=[]  DivideOutMin=[]  DivideOutMax=[]  UdiffTsProdOutMin=[]  UdiffTsProdOutMax=[]  NTsProdOutMin=[]  NTsProdOutMax=[]  UintegralTsProdOutMin=[]  UintegralTsProdOutMax=[]  UngainTsProdOutMin=[]  UngainTsProdOutMax=[]  IntegratorContinuousStateAttributes=''  IntegratorStateMustResolveToSignalObject=off  IntegratorRTWStateStorageClass=Auto  FilterContinuousStateAttributes=''  FilterStateMustResolveToSignalObject=off  FilterRTWStateStorageClass=Auto  ParallelPVariant=Passthrough  IdealPVariant=InternalParameters  IVariant=InternalParameters  DVariant=Disabled  IntegratorVariant=Continuous  SatVariant=Enabled  AWVariant=ContClampingIdeal  PCopyVariant=InternalParamsIdeal  TRVariant=Disabled  FdbkBlocksVariant=Forward  IdealPFdbkVariant=Disabled  SatFdbkVariant=Disabled  DerivativeFilterVariant=Disabled  NVariant=Disabled  NCopyVariant=Disabled_SignalSpec  FilterICVariant=Disabled  IntegratorICVariant=InternalICs  ExternalResetVariant=Disabled  TRSumVariant=Passthrough  SumFdbkVariant=Disabled  SumVariant=Sum_PI  TsampFilterVariant=InternalTs  TsampNgainVariant=Passthrough  TsampIntegralVariant=Passthrough  ExternalSaturationOutDataTypeStr=Inherit: Same as second input
  out_mod_x : Outport
  wires:
  Add/1 -> Data Type Conversion8/1
  actual_Mod_x/1 -> Add/2
  Data Type Conversion8/1 -> PID Controller2/1
  setp_Mod_x/1 -> Add/1
  PID Controller2/1 -> out_mod_x/1

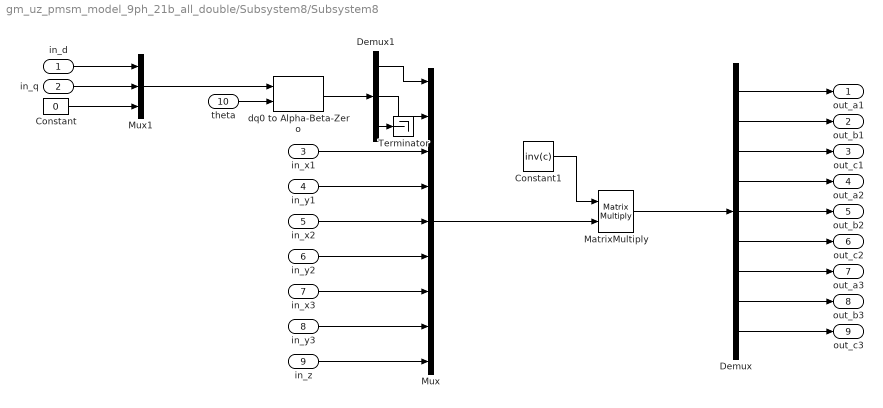
== system gm_uz_pmsm_model_9ph_21b_all_double/Subsystem8/Subsystem8 ==
  in_d : Inport
  in_q : Inport  Port=2
  in_x1 : Inport  Port=3
  in_y1 : Inport  Port=4
  in_x2 : Inport  Port=5
  in_y2 : Inport  Port=6
  in_x3 : Inport  Port=7
  in_y3 : Inport  Port=8
  in_z : Inport  Port=9
  theta : Inport  Port=10
  Constant : Constant  Value=0
  Constant1 : Constant  Value=inv(c)
  Demux : Demux  Outputs=9
  Demux1 : Demux  Outputs=3
  MatrixMultiply : Product  Multiplication=Matrix(*)
  Mux : Mux  Inputs=9
  Mux1 : Mux  Inputs=3
  Terminator : Terminator
  dq0 to Alpha-Beta-Zero : spsdq0toAlphaBetaZeroLib/dq0 to Alpha-Beta-Zero  Alignment=90 degrees behind phase A axis
      settings: SourceProductBaseCode=PS
  out_a1 : Outport
  out_b1 : Outport  Port=2
  out_c1 : Outport  Port=3
  out_a2 : Outport  Port=4
  out_b2 : Outport  Port=5
  out_c2 : Outport  Port=6
  out_a3 : Outport  Port=7
  out_b3 : Outport  Port=8
  out_c3 : Outport  Port=9
  wires:
  Demux/7 -> out_a3/1
  Demux/9 -> out_c3/1
  Demux/8 -> out_b3/1
  Demux/5 -> out_b2/1
  Demux/6 -> out_c2/1
  Demux/4 -> out_a2/1
  Demux/3 -> out_c1/1
  Demux/2 -> out_b1/1
  Constant1/1 -> MatrixMultiply/1
  Demux1/3 -> Terminator/1
  Demux1/2 -> Mux/2
  Demux1/1 -> Mux/1
  dq0 to Alpha-Beta-Zero/1 -> Demux1/1
  theta/1 -> dq0 to Alpha-Beta-Zero/2
  Mux1/1 -> dq0 to Alpha-Beta-Zero/1
  in_d/1 -> Mux1/1
  in_q/1 -> Mux1/2
  Constant/1 -> Mux1/3
  in_z/1 -> Mux/9
  in_x2/1 -> Mux/5
  Mux/1 -> MatrixMultiply/2
  in_y1/1 -> Mux/4
  in_x1/1 -> Mux/3
  Demux/1 -> out_a1/1
  in_y2/1 -> Mux/6
  MatrixMultiply/1 -> Demux/1
  in_y3/1 -> Mux/8
  in_x3/1 -> Mux/7

== system gm_uz_pmsm_model_9ph_21b_all_double/uz_pmsm_model_9ph/Data Type Conversion1 ==
  In1 : Inport
  Data Type Conversion1 : DataTypeConversion  OutDataTypeStr=fixdt(1, 25, 12)  RndMeth=Nearest  SampleTime=1e-08
  Data Type Conversion1_pd1 : Delay  DelayLength=6
  Out1 : Outport
  wires:
  In1/1 -> Data Type Conversion1/1
  Data Type Conversion1/1 -> Data Type Conversion1_pd1/1
  Data Type Conversion1_pd1/1 -> Out1/1

== system gm_uz_pmsm_model_9ph_21b_all_double/uz_pmsm_model_9ph/Data Type Conversion37 ==
  In1 : Inport
  Data Type Conversion37 : DataTypeConversion  OutDataTypeStr=single  RndMeth=Nearest  SampleTime=1e-08
  Data Type Conversion37_pd1 : Delay  DelayLength=6
  Out1 : Outport
  wires:
  In1/1 -> Data Type Conversion37/1
  Data Type Conversion37/1 -> Data Type Conversion37_pd1/1
  Data Type Conversion37_pd1/1 -> Out1/1

== system gm_uz_pmsm_model_9ph_21b_all_double/uz_pmsm_model_9ph/Data Type Conversion5 ==
  In1 : Inport
  Data Type Conversion5 : DataTypeConversion  OutDataTypeStr=single  RndMeth=Nearest  SampleTime=1e-08
  Data Type Conversion5_pd1 : Delay  DelayLength=6
  Out1 : Outport
  wires:
  In1/1 -> Data Type Conversion5/1
  Data Type Conversion5/1 -> Data Type Conversion5_pd1/1
  Data Type Conversion5_pd1/1 -> Out1/1

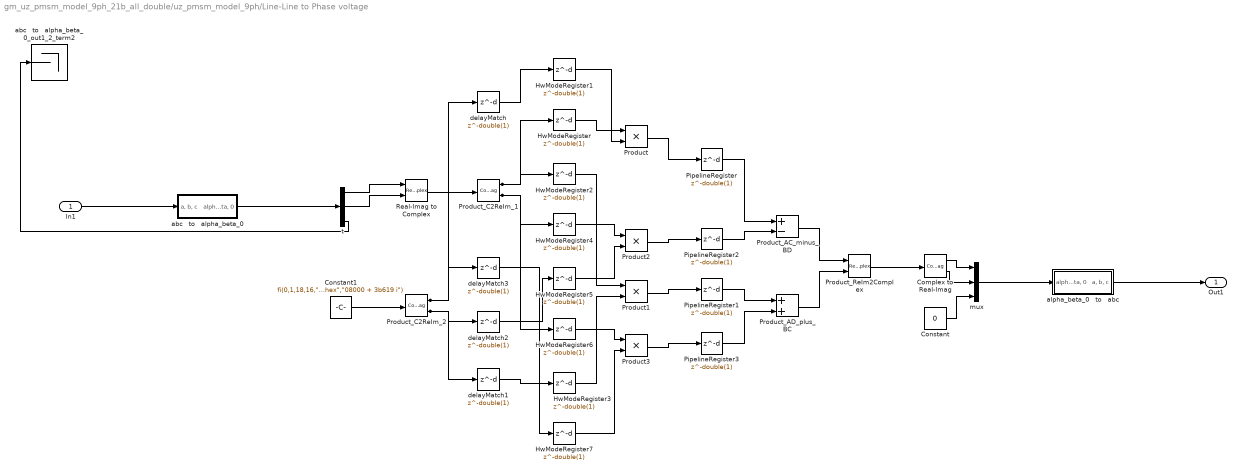
== system gm_uz_pmsm_model_9ph_21b_all_double/uz_pmsm_model_9ph/Line-Line to Phase voltage ==
  In1 : Inport  OutDataTypeStr=fixdt(1, 25, 12)  PortDimensions=[3]  SampleTime=1e-08
  Complex to Real-Imag : ComplexToRealImag  SampleTime=1e-08
  Constant : Constant  Value=0  OutDataTypeStr=fixdt(1, 25, 12)  SampleTime=1e-08
  Constant1 : Constant  Value="fi(0,1,18,16,\"hex\",\"08000 + 3b619 i\")"  OutDataTypeStr=fixdt(1, 18, 16)  SampleTime=1e-08
  HwModeRegister{,1..7} (8 alike) : Delay  DelayLength=double(1)  InitialCondition=0  SampleTime=1e-08
  PipelineRegister{,1..3} (4 alike) : Delay  DelayLength=double(1)  InitialCondition=0  SampleTime=1e-08
  Product{,1..3} (4 alike) : Product  Inputs=**  OutDataTypeStr=fixdt(1, 25, 12)  SampleTime=1e-08
  Product_AC_minus_BD : Sum  Inputs=+-  OutDataTypeStr=fixdt(1, 25, 12)  SampleTime=1e-08
  Product_AD_plus_BC : Sum  OutDataTypeStr=fixdt(1, 25, 12)  SampleTime=1e-08
  Product_C2ReIm_1 : ComplexToRealImag  SampleTime=1e-08
  Product_C2ReIm_2 : ComplexToRealImag  SampleTime=1e-08
  Product_ReIm2Complex : RealImagToComplex  SampleTime=1e-08
  Real-Imag to Complex : RealImagToComplex  ConstantPart="fi(0,1,25,12,\"hex\",\"0000000\")"  SampleTime=1e-08
  abc   to   alpha_beta_0 : Subsystem
  abc   to   alpha_beta_0_out1_2_term2 : Terminator
  alpha_beta_0   to   abc : Subsystem
  delayMatch{,1..3} (4 alike) : Delay  DelayLength=double(1)  InitialCondition=0  SampleTime=1e-08
  mux : Mux  Inputs=3
  t : Demux  Outputs=3
  Out1 : Outport  SampleTime=1e-08
  wires:
  Complex to Real-Imag/1 -> mux/1
  Complex to Real-Imag/2 -> mux/2
  Constant/1 -> mux/3
  Constant1/1 -> Product_C2ReIm_2/1
  mux/1 -> alpha_beta_0   to   abc/1("alpha, beta, 0  ")
  Product_ReIm2Complex/1 -> Complex to Real-Imag/1
  Real-Imag to Complex/1 -> Product_C2ReIm_1/1
  abc   to   alpha_beta_0/1("alpha, beta, 0 ") -> t/1
  alpha_beta_0   to   abc/1("a, b, c") -> Out1/1
  t/1 -> Real-Imag to Complex/1
  t/2 -> Real-Imag to Complex/2
  t/3 -> abc   to   alpha_beta_0_out1_2_term2/1
  Product_C2ReIm_1/1 -> HwModeRegister/1, HwModeRegister2/1
  Product_C2ReIm_1/2 -> HwModeRegister4/1, HwModeRegister6/1
  delayMatch/1 -> HwModeRegister1/1
  delayMatch1/1 -> HwModeRegister3/1
  PipelineRegister/1 -> Product_AC_minus_BD/1
  PipelineRegister1/1 -> Product_AD_plus_BC/1
  PipelineRegister2/1 -> Product_AC_minus_BD/2
  PipelineRegister3/1 -> Product_AD_plus_BC/2
  Product_AC_minus_BD/1 -> Product_ReIm2Complex/1
  Product_AD_plus_BC/1 -> Product_ReIm2Complex/2
  delayMatch3/1 -> HwModeRegister7/1
  delayMatch2/1 -> HwModeRegister5/1
  Product_C2ReIm_2/2 -> delayMatch2/1, delayMatch1/1
  Product_C2ReIm_2/1 -> delayMatch3/1, delayMatch/1
  In1/1 -> abc   to   alpha_beta_0/1("a, b, c")
  Product/1 -> PipelineRegister/1
  HwModeRegister/1 -> Product/1
  HwModeRegister1/1 -> Product/2
  Product1/1 -> PipelineRegister1/1
  HwModeRegister2/1 -> Product1/1
  HwModeRegister3/1 -> Product1/2
  Product2/1 -> PipelineRegister2/1
  HwModeRegister4/1 -> Product2/1
  HwModeRegister5/1 -> Product2/2
  Product3/1 -> PipelineRegister3/1
  HwModeRegister6/1 -> Product3/1
  HwModeRegister7/1 -> Product3/2

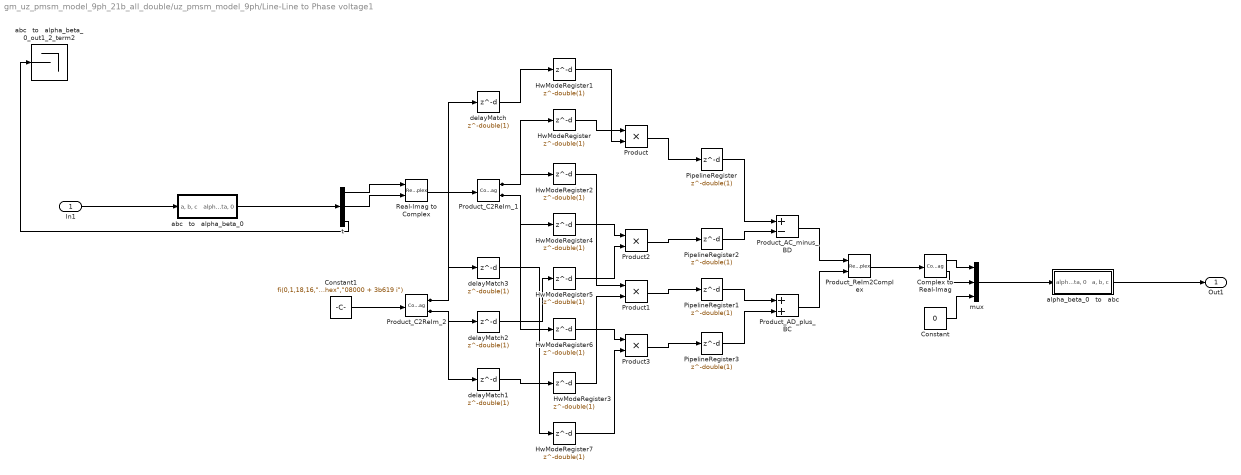
== system gm_uz_pmsm_model_9ph_21b_all_double/uz_pmsm_model_9ph/Line-Line to Phase voltage1 ==
  In1 : Inport  OutDataTypeStr=fixdt(1, 25, 12)  PortDimensions=[3]  SampleTime=1e-08
  Complex to Real-Imag : ComplexToRealImag  SampleTime=1e-08
  Constant : Constant  Value=0  OutDataTypeStr=fixdt(1, 25, 12)  SampleTime=1e-08
  Constant1 : Constant  Value="fi(0,1,18,16,\"hex\",\"08000 + 3b619 i\")"  OutDataTypeStr=fixdt(1, 18, 16)  SampleTime=1e-08
  HwModeRegister{,1..7} (8 alike) : Delay  DelayLength=double(1)  InitialCondition=0  SampleTime=1e-08
  PipelineRegister{,1..3} (4 alike) : Delay  DelayLength=double(1)  InitialCondition=0  SampleTime=1e-08
  Product{,1..3} (4 alike) : Product  Inputs=**  OutDataTypeStr=fixdt(1, 25, 12)  SampleTime=1e-08
  Product_AC_minus_BD : Sum  Inputs=+-  OutDataTypeStr=fixdt(1, 25, 12)  SampleTime=1e-08
  Product_AD_plus_BC : Sum  OutDataTypeStr=fixdt(1, 25, 12)  SampleTime=1e-08
  Product_C2ReIm_1 : ComplexToRealImag  SampleTime=1e-08
  Product_C2ReIm_2 : ComplexToRealImag  SampleTime=1e-08
  Product_ReIm2Complex : RealImagToComplex  SampleTime=1e-08
  Real-Imag to Complex : RealImagToComplex  ConstantPart="fi(0,1,25,12,\"hex\",\"0000000\")"  SampleTime=1e-08
  abc   to   alpha_beta_0 : Subsystem
  abc   to   alpha_beta_0_out1_2_term2 : Terminator
  alpha_beta_0   to   abc : Subsystem
  delayMatch{,1..3} (4 alike) : Delay  DelayLength=double(1)  InitialCondition=0  SampleTime=1e-08
  mux : Mux  Inputs=3
  t : Demux  Outputs=3
  Out1 : Outport  SampleTime=1e-08
  wires:
  Complex to Real-Imag/1 -> mux/1
  Complex to Real-Imag/2 -> mux/2
  Constant/1 -> mux/3
  Constant1/1 -> Product_C2ReIm_2/1
  mux/1 -> alpha_beta_0   to   abc/1("alpha, beta, 0  ")
  Product_ReIm2Complex/1 -> Complex to Real-Imag/1
  Real-Imag to Complex/1 -> Product_C2ReIm_1/1
  abc   to   alpha_beta_0/1("alpha, beta, 0 ") -> t/1
  alpha_beta_0   to   abc/1("a, b, c") -> Out1/1
  t/1 -> Real-Imag to Complex/1
  t/2 -> Real-Imag to Complex/2
  t/3 -> abc   to   alpha_beta_0_out1_2_term2/1
  Product_C2ReIm_1/1 -> HwModeRegister/1, HwModeRegister2/1
  Product_C2ReIm_1/2 -> HwModeRegister4/1, HwModeRegister6/1
  delayMatch/1 -> HwModeRegister1/1
  delayMatch1/1 -> HwModeRegister3/1
  PipelineRegister/1 -> Product_AC_minus_BD/1
  PipelineRegister1/1 -> Product_AD_plus_BC/1
  PipelineRegister2/1 -> Product_AC_minus_BD/2
  PipelineRegister3/1 -> Product_AD_plus_BC/2
  Product_AC_minus_BD/1 -> Product_ReIm2Complex/1
  Product_AD_plus_BC/1 -> Product_ReIm2Complex/2
  delayMatch3/1 -> HwModeRegister7/1
  delayMatch2/1 -> HwModeRegister5/1
  Product_C2ReIm_2/2 -> delayMatch2/1, delayMatch1/1
  Product_C2ReIm_2/1 -> delayMatch3/1, delayMatch/1
  In1/1 -> abc   to   alpha_beta_0/1("a, b, c")
  Product/1 -> PipelineRegister/1
  HwModeRegister/1 -> Product/1
  HwModeRegister1/1 -> Product/2
  Product1/1 -> PipelineRegister1/1
  HwModeRegister2/1 -> Product1/1
  HwModeRegister3/1 -> Product1/2
  Product2/1 -> PipelineRegister2/1
  HwModeRegister4/1 -> Product2/1
  HwModeRegister5/1 -> Product2/2
  Product3/1 -> PipelineRegister3/1
  HwModeRegister6/1 -> Product3/1
  HwModeRegister7/1 -> Product3/2

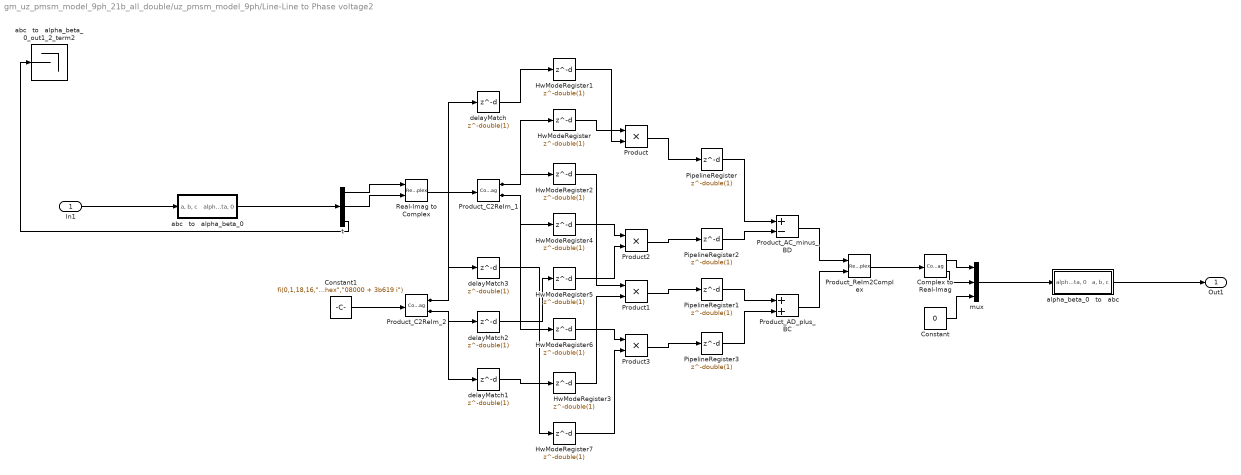
== system gm_uz_pmsm_model_9ph_21b_all_double/uz_pmsm_model_9ph/Line-Line to Phase voltage2 ==
  In1 : Inport  OutDataTypeStr=fixdt(1, 25, 12)  PortDimensions=[3]  SampleTime=1e-08
  Complex to Real-Imag : ComplexToRealImag  SampleTime=1e-08
  Constant : Constant  Value=0  OutDataTypeStr=fixdt(1, 25, 12)  SampleTime=1e-08
  Constant1 : Constant  Value="fi(0,1,18,16,\"hex\",\"08000 + 3b619 i\")"  OutDataTypeStr=fixdt(1, 18, 16)  SampleTime=1e-08
  HwModeRegister{,1..7} (8 alike) : Delay  DelayLength=double(1)  InitialCondition=0  SampleTime=1e-08
  PipelineRegister{,1..3} (4 alike) : Delay  DelayLength=double(1)  InitialCondition=0  SampleTime=1e-08
  Product{,1..3} (4 alike) : Product  Inputs=**  OutDataTypeStr=fixdt(1, 25, 12)  SampleTime=1e-08
  Product_AC_minus_BD : Sum  Inputs=+-  OutDataTypeStr=fixdt(1, 25, 12)  SampleTime=1e-08
  Product_AD_plus_BC : Sum  OutDataTypeStr=fixdt(1, 25, 12)  SampleTime=1e-08
  Product_C2ReIm_1 : ComplexToRealImag  SampleTime=1e-08
  Product_C2ReIm_2 : ComplexToRealImag  SampleTime=1e-08
  Product_ReIm2Complex : RealImagToComplex  SampleTime=1e-08
  Real-Imag to Complex : RealImagToComplex  ConstantPart="fi(0,1,25,12,\"hex\",\"0000000\")"  SampleTime=1e-08
  abc   to   alpha_beta_0 : Subsystem
  abc   to   alpha_beta_0_out1_2_term2 : Terminator
  alpha_beta_0   to   abc : Subsystem
  delayMatch{,1..3} (4 alike) : Delay  DelayLength=double(1)  InitialCondition=0  SampleTime=1e-08
  mux : Mux  Inputs=3
  t : Demux  Outputs=3
  Out1 : Outport  SampleTime=1e-08
  wires:
  Complex to Real-Imag/1 -> mux/1
  Complex to Real-Imag/2 -> mux/2
  Constant/1 -> mux/3
  Constant1/1 -> Product_C2ReIm_2/1
  mux/1 -> alpha_beta_0   to   abc/1("alpha, beta, 0  ")
  Product_ReIm2Complex/1 -> Complex to Real-Imag/1
  Real-Imag to Complex/1 -> Product_C2ReIm_1/1
  abc   to   alpha_beta_0/1("alpha, beta, 0 ") -> t/1
  alpha_beta_0   to   abc/1("a, b, c") -> Out1/1
  t/1 -> Real-Imag to Complex/1
  t/2 -> Real-Imag to Complex/2
  t/3 -> abc   to   alpha_beta_0_out1_2_term2/1
  Product_C2ReIm_1/1 -> HwModeRegister/1, HwModeRegister2/1
  Product_C2ReIm_1/2 -> HwModeRegister4/1, HwModeRegister6/1
  delayMatch/1 -> HwModeRegister1/1
  delayMatch1/1 -> HwModeRegister3/1
  PipelineRegister/1 -> Product_AC_minus_BD/1
  PipelineRegister1/1 -> Product_AD_plus_BC/1
  PipelineRegister2/1 -> Product_AC_minus_BD/2
  PipelineRegister3/1 -> Product_AD_plus_BC/2
  Product_AC_minus_BD/1 -> Product_ReIm2Complex/1
  Product_AD_plus_BC/1 -> Product_ReIm2Complex/2
  delayMatch3/1 -> HwModeRegister7/1
  delayMatch2/1 -> HwModeRegister5/1
  Product_C2ReIm_2/2 -> delayMatch2/1, delayMatch1/1
  Product_C2ReIm_2/1 -> delayMatch3/1, delayMatch/1
  In1/1 -> abc   to   alpha_beta_0/1("a, b, c")
  Product/1 -> PipelineRegister/1
  HwModeRegister/1 -> Product/1
  HwModeRegister1/1 -> Product/2
  Product1/1 -> PipelineRegister1/1
  HwModeRegister2/1 -> Product1/1
  HwModeRegister3/1 -> Product1/2
  Product2/1 -> PipelineRegister2/1
  HwModeRegister4/1 -> Product2/1
  HwModeRegister5/1 -> Product2/2
  Product3/1 -> PipelineRegister3/1
  HwModeRegister6/1 -> Product3/1
  HwModeRegister7/1 -> Product3/2

== system gm_uz_pmsm_model_9ph_21b_all_double/uz_pmsm_model_9ph/Sine_Cosine ==
  In1 : Inport
  Sine_Cosine : Trigonometry  Operator=sincos  SampleTime=1e-08
  Sine_Cosine_pd1 : Delay  DelayLength=27
  Sine_Cosine_pd2 : Delay  DelayLength=27
  Out1 : Outport
  Out2 : Outport  Port=2
  wires:
  In1/1 -> Sine_Cosine/1
  Sine_Cosine/1 -> Sine_Cosine_pd1/1
  Sine_Cosine_pd1/1 -> Out1/1
  Sine_Cosine/2 -> Sine_Cosine_pd2/1
  Sine_Cosine_pd2/1 -> Out2/1
